simulink library "rotation_test_input_library"  (Simulink 8.5)
settings: Solver=ode45  StartTime=0.0  StopTime=10.0  RelTol=1e-3
values from neighbouring files (symbols this model uses):
  A = [0 1 -0.5]'    [rotation_integration_comparison.m]
  f = [10 10 10]'    [rotation_integration_comparison.m]
  rpy_offsets = [0 0 0]'    [rotation_integration_comparison.m]
  rpy_phases = [0 0 0]'    [rotation_integration_comparison.m]
settings Model: Creator=Vorndamme  LastModifiedBy=Vorndamme

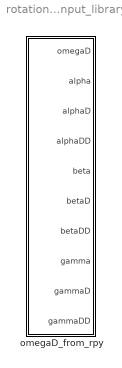
== system rotation_test_input_library ==
  omegaD_from_rpy : Subsystem  mask{A=A, f=f, rpy_offsetts=rpy_offsets, rpy_phases=rpy_phases}
      mask prompts: A "A (Amplitudes)"; f "f (frequency)"; rpy_offsetts "rpy_offsets"

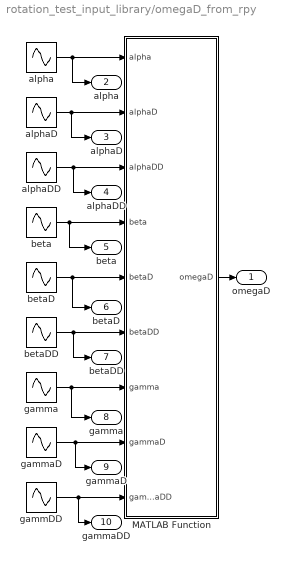
== system rotation_test_input_library/omegaD_from_rpy ==
  MATLAB Function : MATLAB Function  TreatAsAtomicUnit=on
  "alpha " : Sin  Amplitude=A(1)  Bias=rpy_offsets(1)  Frequency=2*pi*f(1)  Phase=rpy_phases(1)  SampleTime=0
  "alphaD " : Sin  Amplitude=2*pi*f(1)*A(1)  Frequency=2*pi*f(1)  Phase=pi/2+rpy_phases(1)  SampleTime=0
  "alphaDD " : Sin  Amplitude=-4*pi^2*f(1)^2*A(1)  Frequency=2*pi*f(1)  Phase=rpy_phases(1)  SampleTime=0
  "beta " : Sin  Amplitude=A(2)  Bias=rpy_offsets(2)  Frequency=2*pi*f(2)  Phase=rpy_phases(2)  SampleTime=0
  "betaD " : Sin  Amplitude=2*pi*f(2)*A(2)  Frequency=2*pi*f(2)  Phase=pi/2+rpy_phases(2)  SampleTime=0
  "betaDD " : Sin  Amplitude=-4*pi^2*f(2)^2*A(2)  Frequency=2*pi*f(2)  Phase=rpy_phases(2)  SampleTime=0
  "gammDD " : Sin  Amplitude=-4*pi^2*f(3)^2*A(3)  Frequency=2*pi*f(3)  Phase=rpy_phases(3)  SampleTime=0
  "gamma  " : Sin  Amplitude=A(3)  Bias=rpy_offsets(3)  Frequency=2*pi*f(3)  Phase=rpy_phases(3)  SampleTime=0
  "gammaD " : Sin  Amplitude=2*pi*f(3)*A(3)  Frequency=2*pi*f(3)  Phase=pi/2+rpy_phases(3)  SampleTime=0
  omegaD : Outport
  alpha : Outport  Port=2
  alphaD : Outport  Port=3
  alphaDD : Outport  Port=4
  beta : Outport  Port=5
  betaD : Outport  Port=6
  betaDD : Outport  Port=7
  gamma : Outport  Port=8
  gammaD : Outport  Port=9
  gammaDD : Outport  Port=10
  wires:
  "alphaD "/1 -> alphaD/1, MATLAB Function/2(alphaD)
  "gammaD "/1 -> gammaD/1, MATLAB Function/8(gammaD)
  "alphaDD "/1 -> alphaDD/1, MATLAB Function/3(alphaDD)
  "betaD "/1 -> betaD/1, MATLAB Function/5(betaD)
  "gammDD "/1 -> gammaDD/1, MATLAB Function/9(gammaDD)
  "beta "/1 -> beta/1, MATLAB Function/4(beta)
  "gamma  "/1 -> gamma/1, MATLAB Function/7(gamma)
  "betaDD "/1 -> betaDD/1, MATLAB Function/6(betaDD)
  "alpha "/1 -> alpha/1, MATLAB Function/1(alpha)
  MATLAB Function/1(omegaD) -> omegaD/1

== matlab function omegaD_from_rpy/MATLAB Function ==
  data: alpha input double; omegaD output double; alphaD input double; alphaDD input double; beta input double; betaD input double; betaDD input double; gamma input double; gammaD input double; gammaDD input double
function omegaD = omegaFromRPY(alpha, alphaD, alphaDD, beta, betaD, betaDD, gamma, gammaD, gammaDD)
%#codegen

omegaD = rpyDD2omegaD([alpha, beta, gamma]', [alphaD, betaD, gammaD]', [alphaDD, betaDD, gammaDD]');
